simulink model "GPESTN1"  (Simulink 6.1)
settings: Solver=ode45  StartTime=0.0  StopTime=1000.0  MaxStep=0.02  MinStep=0.005  RelTol=1e-3
values from neighbouring files (symbols this model uses):
  A_gpe = 2    [data_GPE.m]    (also in data_GPI.m)
  A_stn = 5    [data_GPI.m]    (also in data_STN.m)
  B_gpe = .08    (= 0.08)    [data_GPE.m]    (also in data_GPI.m)
  B_stn = 1    [data_GPI.m]    (also in data_STN.m)
  c_gpe = 1    [data_GPE.m]
  c_stn = 1    [data_STN.m]
  cag0 = i_v_16(177:192)    [launch_sysGPESTN1.m]    (also in launch_sysGPESTN1_GPEDBS.m)
  cas0 = i_v_16(65:80)    [launch_sysGPESTN1.m]    (also in launch_sysGPESTN1_GPEDBS.m)
  egpegpe = -80    [data_synapses.m]
  egpestn = -100    [data_synapses.m]
  ek_gpe = -80.0    (= -80)    [data_GPE.m]
  ek_stn = -80.0    (= -80)    [data_STN.m]
  el_gpe = -55.0    (= -55)    [data_GPE.m]
  el_stn = -60.0    (= -60)    [data_STN.m]
  epsil_gpe = 1*10^-4    (= 0.0001)    [data_GPE.m]
  epsil_stn = 3.75*10^-5    (= 3.75e-05)    [data_STN.m]
  estngpe = 0    [data_synapses.m]
  gahp_gpe = 30.0    (= 30)    [data_GPE.m]
  gahp_stn = 9.0    (= 9)    [data_STN.m]
  gca_gpe = 0.1    [data_GPE.m]
  gca_stn = 0.5    [data_STN.m]
  ggpegpe = .3    (= 0.3)    [data_synapses.m]    (also in launch_sysGPESTN1.m; launch_sysGPESTN1_GPEDBS.m = 0)
  ggpestn = .90    (= 0.9)    [data_synapses.m]
  gk_gpe = 30.0    (= 30)    [data_GPE.m]
  gk_stn = 45.0    (= 45)    [data_STN.m]
  gl_gpe = .1    (= 0.1)    [data_GPE.m]
  gl_stn = 2.25    [data_STN.m]
  gna_gpe = 120    [data_GPE.m]
  gna_stn = 37.5    [data_STN.m]
  gstngpe = .3    (= 0.3)    [data_synapses.m]
  gt_gpe = .5    (= 0.5)    [data_GPE.m]
  gt_stn = 0.5    [data_STN.m]
  hg0 = i_v_16(129:144)    [launch_sysGPESTN1.m]    (also in launch_sysGPESTN1_GPEDBS.m)
  hs0 = i_v_16(17:32)    [launch_sysGPESTN1.m]    (also in launch_sysGPESTN1_GPEDBS.m)
  k1_gpe = 30.0    (= 30)    [data_GPE.m]
  k1_stn = 15.0    (= 15)    [data_STN.m]
  kca_gpe = 15    [data_GPE.m]
  kca_stn = 22.5    [data_STN.m]
  ng0 = i_v_16(145:160)    [launch_sysGPESTN1.m]    (also in launch_sysGPESTN1_GPEDBS.m)
  ns0 = i_v_16(33:48)    [launch_sysGPESTN1.m]    (also in launch_sysGPESTN1_GPEDBS.m)
  phih_gpe = 0.05    [data_GPE.m]
  phih_stn = 0.75    [data_STN.m]
  phin_gpe = 0.1    [data_GPE.m]
  phin_stn = 0.75    [data_STN.m]
  phir_gpe = 1    [data_GPE.m]
  phir_stn = 0.5    [data_STN.m]
  rg0 = i_v_16(161:176)    [launch_sysGPESTN1.m]    (also in launch_sysGPESTN1_GPEDBS.m)
  rs0 = i_v_16(49:64)    [launch_sysGPESTN1.m]    (also in launch_sysGPESTN1_GPEDBS.m)
  sg0 = i_v_16(193:208)    [launch_sysGPESTN1.m]    (also in launch_sysGPESTN1_GPEDBS.m)
  sigmaa_gpe = 2    [data_GPE.m]
  sigmaa_stn = 7.8    [data_STN.m]
  sigmab_stn = -0.07    [data_STN.m]
  sigmagh_gpe = 2.0    (= 2)    [data_GPE.m]
  sigmagh_stn = 8.0    (= 8)    [data_STN.m]
  sigmah_gpe = -12    [data_GPE.m]
  sigmah_stn = -3.1    [data_STN.m]
  sigmam_gpe = 10.0    (= 10)    [data_GPE.m]
  sigmam_stn = 15.0    (= 15)    [data_STN.m]
  sigman_gpe = 14.0    (= 14)    [data_GPE.m]
  sigman_stn = 8.0    (= 8)    [data_STN.m]
  sigmar_gpe = -2.0    (= -2)    [data_GPE.m]
  sigmar_stn = -2.0    (= -2)    [data_STN.m]
  sigmas_gpe = 2    [data_GPE.m]
  sigmas_stn = 8.0    (= 8)    [data_STN.m]
  sigmatauh_gpe = -12    [data_GPE.m]
  sigmatauh_stn = -3.0    (= -3)    [data_STN.m]
  sigmataun_gpe = -12.0    (= -12)    [data_GPE.m]
  sigmataun_stn = -26.0    (= -26)    [data_STN.m]
  sigmataur_stn = -2.2    [data_STN.m]
  ss0 = i_v_16(81:96)    [launch_sysGPESTN1.m]    (also in launch_sysGPESTN1_GPEDBS.m)
  syn_stngpe_gain = .2    (= 0.2)    [data_STN.m]
  tauh0_gpe = .05    (= 0.05)    [data_GPE.m]
  tauh0_stn = 1.0    (= 1)    [data_STN.m]
  tauh1_gpe = .27    (= 0.27)    [data_GPE.m]
  tauh1_stn = 500.0    (= 500)    [data_STN.m]
  taun0_gpe = .05    (= 0.05)    [data_GPE.m]
  taun0_stn = 1.0    (= 1)    [data_STN.m]
  taun1_gpe = .27    (= 0.27)    [data_GPE.m]
  taun1_stn = 100.0    (= 100)    [data_STN.m]
  taur0_stn = 7.1    [data_STN.m]
  taur1_stn = 17.5    [data_STN.m]
  taur_gpe = 30.0    (= 30)    [data_GPE.m]
  theta_gpe = 20    [data_GPE.m]    (also in data_GPI.m)
  theta_stn = 30    [data_GPI.m]    (also in data_STN.m)
  thetaa_gpe = -57.0    (= -57)    [data_GPE.m]
  thetaa_stn = -63.0    (= -63)    [data_STN.m]
  thetab_stn = 0.25    [data_STN.m]
  thetagh_gpe = -57.0    (= -57)    [data_GPE.m]
  thetagh_stn = -39.0    (= -39)    [data_STN.m]
  thetah_gpe = -58.0    (= -58)    [data_GPE.m]
  thetah_stn = -39.0    (= -39)    [data_STN.m]
  thetam_gpe = -37.0    (= -37)    [data_GPE.m]
  thetam_stn = -30.0    (= -30)    [data_STN.m]
  thetan_gpe = -50.0    (= -50)    [data_GPE.m]
  thetan_stn = -32.0    (= -32)    [data_STN.m]
  thetar_gpe = -70.0    (= -70)    [data_GPE.m]
  thetar_stn = -67.0    (= -67)    [data_STN.m]
  thetas_gpe = -35.0    (= -35)    [data_GPE.m]
  thetas_stn = -39.0    (= -39)    [data_STN.m]
  thetatauh_gpe = -40.0    (= -40)    [data_GPE.m]
  thetatauh_stn = -57.0    (= -57)    [data_STN.m]
  thetataun_gpe = -40.0    (= -40)    [data_GPE.m]
  thetataun_stn = -80.0    (= -80)    [data_STN.m]
  thetataur_stn = 68.0    (= 68)    [data_STN.m]
  vg0 = i_v_16(113:128)    [launch_sysGPESTN1.m]    (also in launch_sysGPESTN1_GPEDBS.m)
  vs0 = i_v_16(1:16)    [launch_sysGPESTN1.m]    (also in launch_sysGPESTN1_GPEDBS.m)
undefined symbols (not defined in the file or in its folder): cag01, cas01, hg01, hs01, ng01, ns01, rg01, rs01, sg01, ss01, vg01, vs01
(part 5 of 9)

== system GPESTN1/STN_cell11/Subsystem/iahp ==
  In1 : Inport  Port=1  LatchInput=off
  In2 : Inport  Port=2  LatchInput=off
  In3 : Inport  Port=3  LatchInput=off
  In4 : Inport  Port=4  LatchInput=off
  Fcn : Fcn  Expr=u/(u+k1_stn)
  Fcn1 : Fcn  Expr=(u-ek_stn)*gahp_stn
  Product : Product  SaturateOnIntegerOverflow=on  InputSameDT=on
  Subsystem : Subsystem
  Out1 : Outport
  wires:
  Subsystem/1(Out1) -> Fcn/1
  Fcn1/1 -> Product/2
  Fcn/1 -> Product/1
  In1/1 -> Subsystem/1(In1)
  In2/1 -> Subsystem/2(In2)
  In3/1 -> Fcn1/1
  Product/1 -> Out1/1
  In4/1 -> Subsystem/3(In3)

== system GPESTN1/STN_cell11/Subsystem/ica ==
  In1 : Inport  Orientation=down  Port=1  LatchInput=off
  ica_stn1 : Subsystem
  sinf : Fcn  Expr=1/(1 + exp(-(u-thetas_stn)/sigmas_stn))
  Out1 : Outport
  wires:
  sinf/1 -> ica_stn1/2(In2)
  In1/1 -> sinf/1, ica_stn1/1(In1)
  ica_stn1/1(Out1) -> Out1/1

== system GPESTN1/STN_cell11/Subsystem/ik ==
  In1 : Inport  Port=1  LatchInput=off
  In2 : Inport  Port=2  LatchInput=off
  ik_stn : Subsystem
  n_stn : Subsystem
  Out1 : Outport
  wires:
  n_stn/1(Out1) -> ik_stn/2(In2)
  In1/1 -> ik_stn/1(In1), n_stn/1(In1)
  ik_stn/1(Out1) -> Out1/1
  In2/1 -> n_stn/2(In2)

== system GPESTN1/STN_cell11/Subsystem/ina ==
  In2 : Inport  Port=1  LatchInput=off
  In1 : Inport  Port=2  LatchInput=off
  h_stn : Subsystem
  ina_stn : Subsystem
  minf : Fcn  Expr=1/(1 + exp(-(u-thetam_stn)/sigmam_stn))
  Out1 : Outport
  wires:
  h_stn/1(Out1) -> ina_stn/3(In3)
  minf/1 -> ina_stn/2(In2)
  In2/1 -> minf/1, h_stn/1(In1), ina_stn/1(In1)
  ina_stn/1(Out1) -> Out1/1
  In1/1 -> h_stn/2(In2)

== system GPESTN1/STN_cell11/Subsystem/it ==
  In2 : Inport  Port=1  LatchInput=off
  In1 : Inport  Port=2  LatchInput=off
  ainf : Fcn  Expr=1/(1 + exp(-(u-thetaa_stn)/sigmaa_stn))
  binf : Fcn  Expr=(1/(1 + exp((u-thetab_stn)/sigmab_stn))) - (1/(1 + exp(-thetab_stn/sigmab_stn)))
  it_stn : Subsystem
  r_stn1 : Subsystem
  Out1 : Outport
  wires:
  ainf/1 -> it_stn/3(In3)
  In2/1 -> r_stn1/1(In1), ainf/1, it_stn/1(In1)
  it_stn/1(Out1) -> Out1/1
  r_stn1/1(Out1) -> binf/1
  binf/1 -> it_stn/2(In2)
  In1/1 -> r_stn1/2(In2)

== system GPESTN1/STN_cell12/Subsystem/iahp ==
  In1 : Inport  Port=1  LatchInput=off
  In2 : Inport  Port=2  LatchInput=off
  In3 : Inport  Port=3  LatchInput=off
  In4 : Inport  Port=4  LatchInput=off
  Fcn : Fcn  Expr=u/(u+k1_stn)
  Fcn1 : Fcn  Expr=(u-ek_stn)*gahp_stn
  Product : Product  SaturateOnIntegerOverflow=on  InputSameDT=on
  Subsystem : Subsystem
  Out1 : Outport
  wires:
  Subsystem/1(Out1) -> Fcn/1
  Fcn1/1 -> Product/2
  Fcn/1 -> Product/1
  In1/1 -> Subsystem/1(In1)
  In2/1 -> Subsystem/2(In2)
  In3/1 -> Fcn1/1
  Product/1 -> Out1/1
  In4/1 -> Subsystem/3(In3)

== system GPESTN1/STN_cell12/Subsystem/ica ==
  In1 : Inport  Orientation=down  Port=1  LatchInput=off
  ica_stn1 : Subsystem
  sinf : Fcn  Expr=1/(1 + exp(-(u-thetas_stn)/sigmas_stn))
  Out1 : Outport
  wires:
  sinf/1 -> ica_stn1/2(In2)
  In1/1 -> sinf/1, ica_stn1/1(In1)
  ica_stn1/1(Out1) -> Out1/1

== system GPESTN1/STN_cell12/Subsystem/ik ==
  In1 : Inport  Port=1  LatchInput=off
  In2 : Inport  Port=2  LatchInput=off
  ik_stn : Subsystem
  n_stn : Subsystem
  Out1 : Outport
  wires:
  n_stn/1(Out1) -> ik_stn/2(In2)
  In1/1 -> ik_stn/1(In1), n_stn/1(In1)
  ik_stn/1(Out1) -> Out1/1
  In2/1 -> n_stn/2(In2)

== system GPESTN1/STN_cell12/Subsystem/ina ==
  In2 : Inport  Port=1  LatchInput=off
  In1 : Inport  Port=2  LatchInput=off
  h_stn : Subsystem
  ina_stn : Subsystem
  minf : Fcn  Expr=1/(1 + exp(-(u-thetam_stn)/sigmam_stn))
  Out1 : Outport
  wires:
  h_stn/1(Out1) -> ina_stn/3(In3)
  minf/1 -> ina_stn/2(In2)
  In2/1 -> minf/1, h_stn/1(In1), ina_stn/1(In1)
  ina_stn/1(Out1) -> Out1/1
  In1/1 -> h_stn/2(In2)

== system GPESTN1/STN_cell12/Subsystem/it ==
  In2 : Inport  Port=1  LatchInput=off
  In1 : Inport  Port=2  LatchInput=off
  ainf : Fcn  Expr=1/(1 + exp(-(u-thetaa_stn)/sigmaa_stn))
  binf : Fcn  Expr=(1/(1 + exp((u-thetab_stn)/sigmab_stn))) - (1/(1 + exp(-thetab_stn/sigmab_stn)))
  it_stn : Subsystem
  r_stn1 : Subsystem
  Out1 : Outport
  wires:
  ainf/1 -> it_stn/3(In3)
  In2/1 -> r_stn1/1(In1), ainf/1, it_stn/1(In1)
  it_stn/1(Out1) -> Out1/1
  r_stn1/1(Out1) -> binf/1
  binf/1 -> it_stn/2(In2)
  In1/1 -> r_stn1/2(In2)

== system GPESTN1/STN_cell13/Subsystem/iahp ==
  In1 : Inport  Port=1  LatchInput=off
  In2 : Inport  Port=2  LatchInput=off
  In3 : Inport  Port=3  LatchInput=off
  In4 : Inport  Port=4  LatchInput=off
  Fcn : Fcn  Expr=u/(u+k1_stn)
  Fcn1 : Fcn  Expr=(u-ek_stn)*gahp_stn
  Product : Product  SaturateOnIntegerOverflow=on  InputSameDT=on
  Subsystem : Subsystem
  Out1 : Outport
  wires:
  Subsystem/1(Out1) -> Fcn/1
  Fcn1/1 -> Product/2
  Fcn/1 -> Product/1
  In1/1 -> Subsystem/1(In1)
  In2/1 -> Subsystem/2(In2)
  In3/1 -> Fcn1/1
  Product/1 -> Out1/1
  In4/1 -> Subsystem/3(In3)

== system GPESTN1/STN_cell13/Subsystem/ica ==
  In1 : Inport  Orientation=down  Port=1  LatchInput=off
  ica_stn1 : Subsystem
  sinf : Fcn  Expr=1/(1 + exp(-(u-thetas_stn)/sigmas_stn))
  Out1 : Outport
  wires:
  sinf/1 -> ica_stn1/2(In2)
  In1/1 -> sinf/1, ica_stn1/1(In1)
  ica_stn1/1(Out1) -> Out1/1

== system GPESTN1/STN_cell13/Subsystem/ik ==
  In1 : Inport  Port=1  LatchInput=off
  In2 : Inport  Port=2  LatchInput=off
  ik_stn : Subsystem
  n_stn : Subsystem
  Out1 : Outport
  wires:
  n_stn/1(Out1) -> ik_stn/2(In2)
  In1/1 -> ik_stn/1(In1), n_stn/1(In1)
  ik_stn/1(Out1) -> Out1/1
  In2/1 -> n_stn/2(In2)

== system GPESTN1/STN_cell13/Subsystem/ina ==
  In2 : Inport  Port=1  LatchInput=off
  In1 : Inport  Port=2  LatchInput=off
  h_stn : Subsystem
  ina_stn : Subsystem
  minf : Fcn  Expr=1/(1 + exp(-(u-thetam_stn)/sigmam_stn))
  Out1 : Outport
  wires:
  h_stn/1(Out1) -> ina_stn/3(In3)
  minf/1 -> ina_stn/2(In2)
  In2/1 -> minf/1, h_stn/1(In1), ina_stn/1(In1)
  ina_stn/1(Out1) -> Out1/1
  In1/1 -> h_stn/2(In2)

== system GPESTN1/STN_cell13/Subsystem/it ==
  In2 : Inport  Port=1  LatchInput=off
  In1 : Inport  Port=2  LatchInput=off
  ainf : Fcn  Expr=1/(1 + exp(-(u-thetaa_stn)/sigmaa_stn))
  binf : Fcn  Expr=(1/(1 + exp((u-thetab_stn)/sigmab_stn))) - (1/(1 + exp(-thetab_stn/sigmab_stn)))
  it_stn : Subsystem
  r_stn1 : Subsystem
  Out1 : Outport
  wires:
  ainf/1 -> it_stn/3(In3)
  In2/1 -> r_stn1/1(In1), ainf/1, it_stn/1(In1)
  it_stn/1(Out1) -> Out1/1
  r_stn1/1(Out1) -> binf/1
  binf/1 -> it_stn/2(In2)
  In1/1 -> r_stn1/2(In2)

== system GPESTN1/STN_cell14/Subsystem/iahp ==
  In1 : Inport  Port=1  LatchInput=off
  In2 : Inport  Port=2  LatchInput=off
  In3 : Inport  Port=3  LatchInput=off
  In4 : Inport  Port=4  LatchInput=off
  Fcn : Fcn  Expr=u/(u+k1_stn)
  Fcn1 : Fcn  Expr=(u-ek_stn)*gahp_stn
  Product : Product  SaturateOnIntegerOverflow=on  InputSameDT=on
  Subsystem : Subsystem
  Out1 : Outport
  wires:
  Subsystem/1(Out1) -> Fcn/1
  Fcn1/1 -> Product/2
  Fcn/1 -> Product/1
  In1/1 -> Subsystem/1(In1)
  In2/1 -> Subsystem/2(In2)
  In3/1 -> Fcn1/1
  Product/1 -> Out1/1
  In4/1 -> Subsystem/3(In3)

== system GPESTN1/STN_cell14/Subsystem/ica ==
  In1 : Inport  Orientation=down  Port=1  LatchInput=off
  ica_stn1 : Subsystem
  sinf : Fcn  Expr=1/(1 + exp(-(u-thetas_stn)/sigmas_stn))
  Out1 : Outport
  wires:
  sinf/1 -> ica_stn1/2(In2)
  In1/1 -> sinf/1, ica_stn1/1(In1)
  ica_stn1/1(Out1) -> Out1/1

== system GPESTN1/STN_cell14/Subsystem/ik ==
  In1 : Inport  Port=1  LatchInput=off
  In2 : Inport  Port=2  LatchInput=off
  ik_stn : Subsystem
  n_stn : Subsystem
  Out1 : Outport
  wires:
  n_stn/1(Out1) -> ik_stn/2(In2)
  In1/1 -> ik_stn/1(In1), n_stn/1(In1)
  ik_stn/1(Out1) -> Out1/1
  In2/1 -> n_stn/2(In2)

== system GPESTN1/STN_cell14/Subsystem/ina ==
  In2 : Inport  Port=1  LatchInput=off
  In1 : Inport  Port=2  LatchInput=off
  h_stn : Subsystem
  ina_stn : Subsystem
  minf : Fcn  Expr=1/(1 + exp(-(u-thetam_stn)/sigmam_stn))
  Out1 : Outport
  wires:
  h_stn/1(Out1) -> ina_stn/3(In3)
  minf/1 -> ina_stn/2(In2)
  In2/1 -> minf/1, h_stn/1(In1), ina_stn/1(In1)
  ina_stn/1(Out1) -> Out1/1
  In1/1 -> h_stn/2(In2)

== system GPESTN1/STN_cell14/Subsystem/it ==
  In2 : Inport  Port=1  LatchInput=off
  In1 : Inport  Port=2  LatchInput=off
  ainf : Fcn  Expr=1/(1 + exp(-(u-thetaa_stn)/sigmaa_stn))
  binf : Fcn  Expr=(1/(1 + exp((u-thetab_stn)/sigmab_stn))) - (1/(1 + exp(-thetab_stn/sigmab_stn)))
  it_stn : Subsystem
  r_stn1 : Subsystem
  Out1 : Outport
  wires:
  ainf/1 -> it_stn/3(In3)
  In2/1 -> r_stn1/1(In1), ainf/1, it_stn/1(In1)
  it_stn/1(Out1) -> Out1/1
  r_stn1/1(Out1) -> binf/1
  binf/1 -> it_stn/2(In2)
  In1/1 -> r_stn1/2(In2)

== system GPESTN1/STN_cell15/Subsystem/iahp ==
  In1 : Inport  Port=1  LatchInput=off
  In2 : Inport  Port=2  LatchInput=off
  In3 : Inport  Port=3  LatchInput=off
  In4 : Inport  Port=4  LatchInput=off
  Fcn : Fcn  Expr=u/(u+k1_stn)
  Fcn1 : Fcn  Expr=(u-ek_stn)*gahp_stn
  Product : Product  SaturateOnIntegerOverflow=on  InputSameDT=on
  Subsystem : Subsystem
  Out1 : Outport
  wires:
  Subsystem/1(Out1) -> Fcn/1
  Fcn1/1 -> Product/2
  Fcn/1 -> Product/1
  In1/1 -> Subsystem/1(In1)
  In2/1 -> Subsystem/2(In2)
  In3/1 -> Fcn1/1
  Product/1 -> Out1/1
  In4/1 -> Subsystem/3(In3)

== system GPESTN1/STN_cell15/Subsystem/ica ==
  In1 : Inport  Orientation=down  Port=1  LatchInput=off
  ica_stn1 : Subsystem
  sinf : Fcn  Expr=1/(1 + exp(-(u-thetas_stn)/sigmas_stn))
  Out1 : Outport
  wires:
  sinf/1 -> ica_stn1/2(In2)
  In1/1 -> sinf/1, ica_stn1/1(In1)
  ica_stn1/1(Out1) -> Out1/1

== system GPESTN1/STN_cell15/Subsystem/ik ==
  In1 : Inport  Port=1  LatchInput=off
  In2 : Inport  Port=2  LatchInput=off
  ik_stn : Subsystem
  n_stn : Subsystem
  Out1 : Outport
  wires:
  n_stn/1(Out1) -> ik_stn/2(In2)
  In1/1 -> ik_stn/1(In1), n_stn/1(In1)
  ik_stn/1(Out1) -> Out1/1
  In2/1 -> n_stn/2(In2)

== system GPESTN1/STN_cell15/Subsystem/ina ==
  In2 : Inport  Port=1  LatchInput=off
  In1 : Inport  Port=2  LatchInput=off
  h_stn : Subsystem
  ina_stn : Subsystem
  minf : Fcn  Expr=1/(1 + exp(-(u-thetam_stn)/sigmam_stn))
  Out1 : Outport
  wires:
  h_stn/1(Out1) -> ina_stn/3(In3)
  minf/1 -> ina_stn/2(In2)
  In2/1 -> minf/1, h_stn/1(In1), ina_stn/1(In1)
  ina_stn/1(Out1) -> Out1/1
  In1/1 -> h_stn/2(In2)

== system GPESTN1/STN_cell15/Subsystem/it ==
  In2 : Inport  Port=1  LatchInput=off
  In1 : Inport  Port=2  LatchInput=off
  ainf : Fcn  Expr=1/(1 + exp(-(u-thetaa_stn)/sigmaa_stn))
  binf : Fcn  Expr=(1/(1 + exp((u-thetab_stn)/sigmab_stn))) - (1/(1 + exp(-thetab_stn/sigmab_stn)))
  it_stn : Subsystem
  r_stn1 : Subsystem
  Out1 : Outport
  wires:
  ainf/1 -> it_stn/3(In3)
  In2/1 -> r_stn1/1(In1), ainf/1, it_stn/1(In1)
  it_stn/1(Out1) -> Out1/1
  r_stn1/1(Out1) -> binf/1
  binf/1 -> it_stn/2(In2)
  In1/1 -> r_stn1/2(In2)

== system GPESTN1/STN_cell16/Subsystem/iahp ==
  In1 : Inport  Port=1  LatchInput=off
  In2 : Inport  Port=2  LatchInput=off
  In3 : Inport  Port=3  LatchInput=off
  In4 : Inport  Port=4  LatchInput=off
  Fcn : Fcn  Expr=u/(u+k1_stn)
  Fcn1 : Fcn  Expr=(u-ek_stn)*gahp_stn
  Product : Product  SaturateOnIntegerOverflow=on  InputSameDT=on
  Subsystem : Subsystem
  Out1 : Outport
  wires:
  Subsystem/1(Out1) -> Fcn/1
  Fcn1/1 -> Product/2
  Fcn/1 -> Product/1
  In1/1 -> Subsystem/1(In1)
  In2/1 -> Subsystem/2(In2)
  In3/1 -> Fcn1/1
  Product/1 -> Out1/1
  In4/1 -> Subsystem/3(In3)

== system GPESTN1/STN_cell16/Subsystem/ica ==
  In1 : Inport  Orientation=down  Port=1  LatchInput=off
  ica_stn1 : Subsystem
  sinf : Fcn  Expr=1/(1 + exp(-(u-thetas_stn)/sigmas_stn))
  Out1 : Outport
  wires:
  sinf/1 -> ica_stn1/2(In2)
  In1/1 -> sinf/1, ica_stn1/1(In1)
  ica_stn1/1(Out1) -> Out1/1

== system GPESTN1/STN_cell16/Subsystem/ik ==
  In1 : Inport  Port=1  LatchInput=off
  In2 : Inport  Port=2  LatchInput=off
  ik_stn : Subsystem
  n_stn : Subsystem
  Out1 : Outport
  wires:
  n_stn/1(Out1) -> ik_stn/2(In2)
  In1/1 -> ik_stn/1(In1), n_stn/1(In1)
  ik_stn/1(Out1) -> Out1/1
  In2/1 -> n_stn/2(In2)

== system GPESTN1/STN_cell16/Subsystem/ina ==
  In2 : Inport  Port=1  LatchInput=off
  In1 : Inport  Port=2  LatchInput=off
  h_stn : Subsystem
  ina_stn : Subsystem
  minf : Fcn  Expr=1/(1 + exp(-(u-thetam_stn)/sigmam_stn))
  Out1 : Outport
  wires:
  h_stn/1(Out1) -> ina_stn/3(In3)
  minf/1 -> ina_stn/2(In2)
  In2/1 -> minf/1, h_stn/1(In1), ina_stn/1(In1)
  ina_stn/1(Out1) -> Out1/1
  In1/1 -> h_stn/2(In2)

== system GPESTN1/STN_cell16/Subsystem/it ==
  In2 : Inport  Port=1  LatchInput=off
  In1 : Inport  Port=2  LatchInput=off
  ainf : Fcn  Expr=1/(1 + exp(-(u-thetaa_stn)/sigmaa_stn))
  binf : Fcn  Expr=(1/(1 + exp((u-thetab_stn)/sigmab_stn))) - (1/(1 + exp(-thetab_stn/sigmab_stn)))
  it_stn : Subsystem
  r_stn1 : Subsystem
  Out1 : Outport
  wires:
  ainf/1 -> it_stn/3(In3)
  In2/1 -> r_stn1/1(In1), ainf/1, it_stn/1(In1)
  it_stn/1(Out1) -> Out1/1
  r_stn1/1(Out1) -> binf/1
  binf/1 -> it_stn/2(In2)
  In1/1 -> r_stn1/2(In2)

== system GPESTN1/STN_cell17/Subsystem/iahp ==
  In1 : Inport  Port=1  LatchInput=off
  In2 : Inport  Port=2  LatchInput=off
  In3 : Inport  Port=3  LatchInput=off
  In4 : Inport  Port=4  LatchInput=off
  Fcn : Fcn  Expr=u/(u+k1_stn)
  Fcn1 : Fcn  Expr=(u-ek_stn)*gahp_stn
  Product : Product  SaturateOnIntegerOverflow=on  InputSameDT=on
  Subsystem : Subsystem
  Out1 : Outport
  wires:
  Subsystem/1(Out1) -> Fcn/1
  Fcn1/1 -> Product/2
  Fcn/1 -> Product/1
  In1/1 -> Subsystem/1(In1)
  In2/1 -> Subsystem/2(In2)
  In3/1 -> Fcn1/1
  Product/1 -> Out1/1
  In4/1 -> Subsystem/3(In3)

== system GPESTN1/STN_cell17/Subsystem/ica ==
  In1 : Inport  Orientation=down  Port=1  LatchInput=off
  ica_stn1 : Subsystem
  sinf : Fcn  Expr=1/(1 + exp(-(u-thetas_stn)/sigmas_stn))
  Out1 : Outport
  wires:
  sinf/1 -> ica_stn1/2(In2)
  In1/1 -> sinf/1, ica_stn1/1(In1)
  ica_stn1/1(Out1) -> Out1/1

== system GPESTN1/STN_cell17/Subsystem/ik ==
  In1 : Inport  Port=1  LatchInput=off
  In2 : Inport  Port=2  LatchInput=off
  ik_stn : Subsystem
  n_stn : Subsystem
  Out1 : Outport
  wires:
  n_stn/1(Out1) -> ik_stn/2(In2)
  In1/1 -> ik_stn/1(In1), n_stn/1(In1)
  ik_stn/1(Out1) -> Out1/1
  In2/1 -> n_stn/2(In2)

== system GPESTN1/STN_cell17/Subsystem/ina ==
  In2 : Inport  Port=1  LatchInput=off
  In1 : Inport  Port=2  LatchInput=off
  h_stn : Subsystem
  ina_stn : Subsystem
  minf : Fcn  Expr=1/(1 + exp(-(u-thetam_stn)/sigmam_stn))
  Out1 : Outport
  wires:
  h_stn/1(Out1) -> ina_stn/3(In3)
  minf/1 -> ina_stn/2(In2)
  In2/1 -> minf/1, h_stn/1(In1), ina_stn/1(In1)
  ina_stn/1(Out1) -> Out1/1
  In1/1 -> h_stn/2(In2)

== system GPESTN1/STN_cell17/Subsystem/it ==
  In2 : Inport  Port=1  LatchInput=off
  In1 : Inport  Port=2  LatchInput=off
  ainf : Fcn  Expr=1/(1 + exp(-(u-thetaa_stn)/sigmaa_stn))
  binf : Fcn  Expr=(1/(1 + exp((u-thetab_stn)/sigmab_stn))) - (1/(1 + exp(-thetab_stn/sigmab_stn)))
  it_stn : Subsystem
  r_stn1 : Subsystem
  Out1 : Outport
  wires:
  ainf/1 -> it_stn/3(In3)
  In2/1 -> r_stn1/1(In1), ainf/1, it_stn/1(In1)
  it_stn/1(Out1) -> Out1/1
  r_stn1/1(Out1) -> binf/1
  binf/1 -> it_stn/2(In2)
  In1/1 -> r_stn1/2(In2)

== system GPESTN1/STN_cell2/Subsystem/iahp ==
  In1 : Inport  Port=1  LatchInput=off
  In2 : Inport  Port=2  LatchInput=off
  In3 : Inport  Port=3  LatchInput=off
  In4 : Inport  Port=4  LatchInput=off
  Fcn : Fcn  Expr=u/(u+k1_stn)
  Fcn1 : Fcn  Expr=(u-ek_stn)*gahp_stn
  Product : Product  SaturateOnIntegerOverflow=on  InputSameDT=on
  Subsystem : Subsystem
  Out1 : Outport
  wires:
  Subsystem/1(Out1) -> Fcn/1
  Fcn1/1 -> Product/2
  Fcn/1 -> Product/1
  In1/1 -> Subsystem/1(In1)
  In2/1 -> Subsystem/2(In2)
  In3/1 -> Fcn1/1
  Product/1 -> Out1/1
  In4/1 -> Subsystem/3(In3)

== system GPESTN1/STN_cell2/Subsystem/ica ==
  In1 : Inport  Orientation=down  Port=1  LatchInput=off
  ica_stn1 : Subsystem
  sinf : Fcn  Expr=1/(1 + exp(-(u-thetas_stn)/sigmas_stn))
  Out1 : Outport
  wires:
  sinf/1 -> ica_stn1/2(In2)
  In1/1 -> sinf/1, ica_stn1/1(In1)
  ica_stn1/1(Out1) -> Out1/1

== system GPESTN1/STN_cell2/Subsystem/ik ==
  In1 : Inport  Port=1  LatchInput=off
  In2 : Inport  Port=2  LatchInput=off
  ik_stn : Subsystem
  n_stn : Subsystem
  Out1 : Outport
  wires:
  n_stn/1(Out1) -> ik_stn/2(In2)
  In1/1 -> ik_stn/1(In1), n_stn/1(In1)
  ik_stn/1(Out1) -> Out1/1
  In2/1 -> n_stn/2(In2)

== system GPESTN1/STN_cell2/Subsystem/ina ==
  In2 : Inport  Port=1  LatchInput=off
  In1 : Inport  Port=2  LatchInput=off
  h_stn : Subsystem
  ina_stn : Subsystem
  minf : Fcn  Expr=1/(1 + exp(-(u-thetam_stn)/sigmam_stn))
  Out1 : Outport
  wires:
  h_stn/1(Out1) -> ina_stn/3(In3)
  minf/1 -> ina_stn/2(In2)
  In2/1 -> minf/1, h_stn/1(In1), ina_stn/1(In1)
  ina_stn/1(Out1) -> Out1/1
  In1/1 -> h_stn/2(In2)

== system GPESTN1/STN_cell2/Subsystem/it ==
  In2 : Inport  Port=1  LatchInput=off
  In1 : Inport  Port=2  LatchInput=off
  ainf : Fcn  Expr=1/(1 + exp(-(u-thetaa_stn)/sigmaa_stn))
  binf : Fcn  Expr=(1/(1 + exp((u-thetab_stn)/sigmab_stn))) - (1/(1 + exp(-thetab_stn/sigmab_stn)))
  it_stn : Subsystem
  r_stn1 : Subsystem
  Out1 : Outport
  wires:
  ainf/1 -> it_stn/3(In3)
  In2/1 -> r_stn1/1(In1), ainf/1, it_stn/1(In1)
  it_stn/1(Out1) -> Out1/1
  r_stn1/1(Out1) -> binf/1
  binf/1 -> it_stn/2(In2)
  In1/1 -> r_stn1/2(In2)

== system GPESTN1/STN_cell3/Subsystem/iahp ==
  In1 : Inport  Port=1  LatchInput=off
  In2 : Inport  Port=2  LatchInput=off
  In3 : Inport  Port=3  LatchInput=off
  In4 : Inport  Port=4  LatchInput=off
  Fcn : Fcn  Expr=u/(u+k1_stn)
  Fcn1 : Fcn  Expr=(u-ek_stn)*gahp_stn
  Product : Product  SaturateOnIntegerOverflow=on  InputSameDT=on
  Subsystem : Subsystem
  Out1 : Outport
  wires:
  Subsystem/1(Out1) -> Fcn/1
  Fcn1/1 -> Product/2
  Fcn/1 -> Product/1
  In1/1 -> Subsystem/1(In1)
  In2/1 -> Subsystem/2(In2)
  In3/1 -> Fcn1/1
  Product/1 -> Out1/1
  In4/1 -> Subsystem/3(In3)

== system GPESTN1/STN_cell3/Subsystem/ica ==
  In1 : Inport  Orientation=down  Port=1  LatchInput=off
  ica_stn1 : Subsystem
  sinf : Fcn  Expr=1/(1 + exp(-(u-thetas_stn)/sigmas_stn))
  Out1 : Outport
  wires:
  sinf/1 -> ica_stn1/2(In2)
  In1/1 -> sinf/1, ica_stn1/1(In1)
  ica_stn1/1(Out1) -> Out1/1

== system GPESTN1/STN_cell3/Subsystem/ik ==
  In1 : Inport  Port=1  LatchInput=off
  In2 : Inport  Port=2  LatchInput=off
  ik_stn : Subsystem
  n_stn : Subsystem
  Out1 : Outport
  wires:
  n_stn/1(Out1) -> ik_stn/2(In2)
  In1/1 -> ik_stn/1(In1), n_stn/1(In1)
  ik_stn/1(Out1) -> Out1/1
  In2/1 -> n_stn/2(In2)

== system GPESTN1/STN_cell3/Subsystem/ina ==
  In2 : Inport  Port=1  LatchInput=off
  In1 : Inport  Port=2  LatchInput=off
  h_stn : Subsystem
  ina_stn : Subsystem
  minf : Fcn  Expr=1/(1 + exp(-(u-thetam_stn)/sigmam_stn))
  Out1 : Outport
  wires:
  h_stn/1(Out1) -> ina_stn/3(In3)
  minf/1 -> ina_stn/2(In2)
  In2/1 -> minf/1, h_stn/1(In1), ina_stn/1(In1)
  ina_stn/1(Out1) -> Out1/1
  In1/1 -> h_stn/2(In2)

== system GPESTN1/STN_cell3/Subsystem/it ==
  In2 : Inport  Port=1  LatchInput=off
  In1 : Inport  Port=2  LatchInput=off
  ainf : Fcn  Expr=1/(1 + exp(-(u-thetaa_stn)/sigmaa_stn))
  binf : Fcn  Expr=(1/(1 + exp((u-thetab_stn)/sigmab_stn))) - (1/(1 + exp(-thetab_stn/sigmab_stn)))
  it_stn : Subsystem
  r_stn1 : Subsystem
  Out1 : Outport
  wires:
  ainf/1 -> it_stn/3(In3)
  In2/1 -> r_stn1/1(In1), ainf/1, it_stn/1(In1)
  it_stn/1(Out1) -> Out1/1
  r_stn1/1(Out1) -> binf/1
  binf/1 -> it_stn/2(In2)
  In1/1 -> r_stn1/2(In2)

== system GPESTN1/STN_cell5/Subsystem/iahp ==
  In1 : Inport  Port=1  LatchInput=off
  In2 : Inport  Port=2  LatchInput=off
  In3 : Inport  Port=3  LatchInput=off
  In4 : Inport  Port=4  LatchInput=off
  Fcn : Fcn  Expr=u/(u+k1_stn)
  Fcn1 : Fcn  Expr=(u-ek_stn)*gahp_stn
  Product : Product  SaturateOnIntegerOverflow=on  InputSameDT=on
  Subsystem : Subsystem
  Out1 : Outport
  wires:
  Subsystem/1(Out1) -> Fcn/1
  Fcn1/1 -> Product/2
  Fcn/1 -> Product/1
  In1/1 -> Subsystem/1(In1)
  In2/1 -> Subsystem/2(In2)
  In3/1 -> Fcn1/1
  Product/1 -> Out1/1
  In4/1 -> Subsystem/3(In3)

== system GPESTN1/STN_cell5/Subsystem/ica ==
  In1 : Inport  Orientation=down  Port=1  LatchInput=off
  ica_stn1 : Subsystem
  sinf : Fcn  Expr=1/(1 + exp(-(u-thetas_stn)/sigmas_stn))
  Out1 : Outport
  wires:
  sinf/1 -> ica_stn1/2(In2)
  In1/1 -> sinf/1, ica_stn1/1(In1)
  ica_stn1/1(Out1) -> Out1/1

== system GPESTN1/STN_cell5/Subsystem/ik ==
  In1 : Inport  Port=1  LatchInput=off
  In2 : Inport  Port=2  LatchInput=off
  ik_stn : Subsystem
  n_stn : Subsystem
  Out1 : Outport
  wires:
  n_stn/1(Out1) -> ik_stn/2(In2)
  In1/1 -> ik_stn/1(In1), n_stn/1(In1)
  ik_stn/1(Out1) -> Out1/1
  In2/1 -> n_stn/2(In2)

== system GPESTN1/STN_cell5/Subsystem/ina ==
  In2 : Inport  Port=1  LatchInput=off
  In1 : Inport  Port=2  LatchInput=off
  h_stn : Subsystem
  ina_stn : Subsystem
  minf : Fcn  Expr=1/(1 + exp(-(u-thetam_stn)/sigmam_stn))
  Out1 : Outport
  wires:
  h_stn/1(Out1) -> ina_stn/3(In3)
  minf/1 -> ina_stn/2(In2)
  In2/1 -> minf/1, h_stn/1(In1), ina_stn/1(In1)
  ina_stn/1(Out1) -> Out1/1
  In1/1 -> h_stn/2(In2)

== system GPESTN1/STN_cell5/Subsystem/it ==
  In2 : Inport  Port=1  LatchInput=off
  In1 : Inport  Port=2  LatchInput=off
  ainf : Fcn  Expr=1/(1 + exp(-(u-thetaa_stn)/sigmaa_stn))
  binf : Fcn  Expr=(1/(1 + exp((u-thetab_stn)/sigmab_stn))) - (1/(1 + exp(-thetab_stn/sigmab_stn)))
  it_stn : Subsystem
  r_stn1 : Subsystem
  Out1 : Outport
  wires:
  ainf/1 -> it_stn/3(In3)
  In2/1 -> r_stn1/1(In1), ainf/1, it_stn/1(In1)
  it_stn/1(Out1) -> Out1/1
  r_stn1/1(Out1) -> binf/1
  binf/1 -> it_stn/2(In2)
  In1/1 -> r_stn1/2(In2)

== system GPESTN1/STN_cell6/Subsystem/iahp ==
  In1 : Inport  Port=1  LatchInput=off
  In2 : Inport  Port=2  LatchInput=off
  In3 : Inport  Port=3  LatchInput=off
  In4 : Inport  Port=4  LatchInput=off
  Fcn : Fcn  Expr=u/(u+k1_stn)
  Fcn1 : Fcn  Expr=(u-ek_stn)*gahp_stn
  Product : Product  SaturateOnIntegerOverflow=on  InputSameDT=on
  Subsystem : Subsystem
  Out1 : Outport
  wires:
  Subsystem/1(Out1) -> Fcn/1
  Fcn1/1 -> Product/2
  Fcn/1 -> Product/1
  In1/1 -> Subsystem/1(In1)
  In2/1 -> Subsystem/2(In2)
  In3/1 -> Fcn1/1
  Product/1 -> Out1/1
  In4/1 -> Subsystem/3(In3)

== system GPESTN1/STN_cell6/Subsystem/ica ==
  In1 : Inport  Orientation=down  Port=1  LatchInput=off
  ica_stn1 : Subsystem
  sinf : Fcn  Expr=1/(1 + exp(-(u-thetas_stn)/sigmas_stn))
  Out1 : Outport
  wires:
  sinf/1 -> ica_stn1/2(In2)
  In1/1 -> sinf/1, ica_stn1/1(In1)
  ica_stn1/1(Out1) -> Out1/1

== system GPESTN1/STN_cell6/Subsystem/ik ==
  In1 : Inport  Port=1  LatchInput=off
  In2 : Inport  Port=2  LatchInput=off
  ik_stn : Subsystem
  n_stn : Subsystem
  Out1 : Outport
  wires:
  n_stn/1(Out1) -> ik_stn/2(In2)
  In1/1 -> ik_stn/1(In1), n_stn/1(In1)
  ik_stn/1(Out1) -> Out1/1
  In2/1 -> n_stn/2(In2)

== system GPESTN1/STN_cell6/Subsystem/ina ==
  In2 : Inport  Port=1  LatchInput=off
  In1 : Inport  Port=2  LatchInput=off
  h_stn : Subsystem
  ina_stn : Subsystem
  minf : Fcn  Expr=1/(1 + exp(-(u-thetam_stn)/sigmam_stn))
  Out1 : Outport
  wires:
  h_stn/1(Out1) -> ina_stn/3(In3)
  minf/1 -> ina_stn/2(In2)
  In2/1 -> minf/1, h_stn/1(In1), ina_stn/1(In1)
  ina_stn/1(Out1) -> Out1/1
  In1/1 -> h_stn/2(In2)

== system GPESTN1/STN_cell6/Subsystem/it ==
  In2 : Inport  Port=1  LatchInput=off
  In1 : Inport  Port=2  LatchInput=off
  ainf : Fcn  Expr=1/(1 + exp(-(u-thetaa_stn)/sigmaa_stn))
  binf : Fcn  Expr=(1/(1 + exp((u-thetab_stn)/sigmab_stn))) - (1/(1 + exp(-thetab_stn/sigmab_stn)))
  it_stn : Subsystem
  r_stn1 : Subsystem
  Out1 : Outport
  wires:
  ainf/1 -> it_stn/3(In3)
  In2/1 -> r_stn1/1(In1), ainf/1, it_stn/1(In1)
  it_stn/1(Out1) -> Out1/1
  r_stn1/1(Out1) -> binf/1
  binf/1 -> it_stn/2(In2)
  In1/1 -> r_stn1/2(In2)

== system GPESTN1/STN_cell7/Subsystem/iahp ==
  In1 : Inport  Port=1  LatchInput=off
  In2 : Inport  Port=2  LatchInput=off
  In3 : Inport  Port=3  LatchInput=off
  In4 : Inport  Port=4  LatchInput=off
  Fcn : Fcn  Expr=u/(u+k1_stn)
  Fcn1 : Fcn  Expr=(u-ek_stn)*gahp_stn
  Product : Product  SaturateOnIntegerOverflow=on  InputSameDT=on
  Subsystem : Subsystem
  Out1 : Outport
  wires:
  Subsystem/1(Out1) -> Fcn/1
  Fcn1/1 -> Product/2
  Fcn/1 -> Product/1
  In1/1 -> Subsystem/1(In1)
  In2/1 -> Subsystem/2(In2)
  In3/1 -> Fcn1/1
  Product/1 -> Out1/1
  In4/1 -> Subsystem/3(In3)

== system GPESTN1/STN_cell7/Subsystem/ica ==
  In1 : Inport  Orientation=down  Port=1  LatchInput=off
  ica_stn1 : Subsystem
  sinf : Fcn  Expr=1/(1 + exp(-(u-thetas_stn)/sigmas_stn))
  Out1 : Outport
  wires:
  sinf/1 -> ica_stn1/2(In2)
  In1/1 -> sinf/1, ica_stn1/1(In1)
  ica_stn1/1(Out1) -> Out1/1

== system GPESTN1/STN_cell7/Subsystem/ik ==
  In1 : Inport  Port=1  LatchInput=off
  In2 : Inport  Port=2  LatchInput=off
  ik_stn : Subsystem
  n_stn : Subsystem
  Out1 : Outport
  wires:
  n_stn/1(Out1) -> ik_stn/2(In2)
  In1/1 -> ik_stn/1(In1), n_stn/1(In1)
  ik_stn/1(Out1) -> Out1/1
  In2/1 -> n_stn/2(In2)

== system GPESTN1/STN_cell7/Subsystem/ina ==
  In2 : Inport  Port=1  LatchInput=off
  In1 : Inport  Port=2  LatchInput=off
  h_stn : Subsystem
  ina_stn : Subsystem
  minf : Fcn  Expr=1/(1 + exp(-(u-thetam_stn)/sigmam_stn))
  Out1 : Outport
  wires:
  h_stn/1(Out1) -> ina_stn/3(In3)
  minf/1 -> ina_stn/2(In2)
  In2/1 -> minf/1, h_stn/1(In1), ina_stn/1(In1)
  ina_stn/1(Out1) -> Out1/1
  In1/1 -> h_stn/2(In2)

== system GPESTN1/STN_cell7/Subsystem/it ==
  In2 : Inport  Port=1  LatchInput=off
  In1 : Inport  Port=2  LatchInput=off
  ainf : Fcn  Expr=1/(1 + exp(-(u-thetaa_stn)/sigmaa_stn))
  binf : Fcn  Expr=(1/(1 + exp((u-thetab_stn)/sigmab_stn))) - (1/(1 + exp(-thetab_stn/sigmab_stn)))
  it_stn : Subsystem
  r_stn1 : Subsystem
  Out1 : Outport
  wires:
  ainf/1 -> it_stn/3(In3)
  In2/1 -> r_stn1/1(In1), ainf/1, it_stn/1(In1)
  it_stn/1(Out1) -> Out1/1
  r_stn1/1(Out1) -> binf/1
  binf/1 -> it_stn/2(In2)
  In1/1 -> r_stn1/2(In2)

== system GPESTN1/STN_cell8/Subsystem/iahp ==
  In1 : Inport  Port=1  LatchInput=off
  In2 : Inport  Port=2  LatchInput=off
  In3 : Inport  Port=3  LatchInput=off
  In4 : Inport  Port=4  LatchInput=off
  Fcn : Fcn  Expr=u/(u+k1_stn)
  Fcn1 : Fcn  Expr=(u-ek_stn)*gahp_stn
  Product : Product  SaturateOnIntegerOverflow=on  InputSameDT=on
  Subsystem : Subsystem
  Out1 : Outport
  wires:
  Subsystem/1(Out1) -> Fcn/1
  Fcn1/1 -> Product/2
  Fcn/1 -> Product/1
  In1/1 -> Subsystem/1(In1)
  In2/1 -> Subsystem/2(In2)
  In3/1 -> Fcn1/1
  Product/1 -> Out1/1
  In4/1 -> Subsystem/3(In3)

== system GPESTN1/STN_cell8/Subsystem/ica ==
  In1 : Inport  Orientation=down  Port=1  LatchInput=off
  ica_stn1 : Subsystem
  sinf : Fcn  Expr=1/(1 + exp(-(u-thetas_stn)/sigmas_stn))
  Out1 : Outport
  wires:
  sinf/1 -> ica_stn1/2(In2)
  In1/1 -> sinf/1, ica_stn1/1(In1)
  ica_stn1/1(Out1) -> Out1/1

== system GPESTN1/STN_cell8/Subsystem/ik ==
  In1 : Inport  Port=1  LatchInput=off
  In2 : Inport  Port=2  LatchInput=off
  ik_stn : Subsystem
  n_stn : Subsystem
  Out1 : Outport
  wires:
  n_stn/1(Out1) -> ik_stn/2(In2)
  In1/1 -> ik_stn/1(In1), n_stn/1(In1)
  ik_stn/1(Out1) -> Out1/1
  In2/1 -> n_stn/2(In2)

== system GPESTN1/STN_cell8/Subsystem/ina ==
  In2 : Inport  Port=1  LatchInput=off
  In1 : Inport  Port=2  LatchInput=off
  h_stn : Subsystem
  ina_stn : Subsystem
  minf : Fcn  Expr=1/(1 + exp(-(u-thetam_stn)/sigmam_stn))
  Out1 : Outport
  wires:
  h_stn/1(Out1) -> ina_stn/3(In3)
  minf/1 -> ina_stn/2(In2)
  In2/1 -> minf/1, h_stn/1(In1), ina_stn/1(In1)
  ina_stn/1(Out1) -> Out1/1
  In1/1 -> h_stn/2(In2)

== system GPESTN1/STN_cell8/Subsystem/it ==
  In2 : Inport  Port=1  LatchInput=off
  In1 : Inport  Port=2  LatchInput=off
  ainf : Fcn  Expr=1/(1 + exp(-(u-thetaa_stn)/sigmaa_stn))
  binf : Fcn  Expr=(1/(1 + exp((u-thetab_stn)/sigmab_stn))) - (1/(1 + exp(-thetab_stn/sigmab_stn)))
  it_stn : Subsystem
  r_stn1 : Subsystem
  Out1 : Outport
  wires:
  ainf/1 -> it_stn/3(In3)
  In2/1 -> r_stn1/1(In1), ainf/1, it_stn/1(In1)
  it_stn/1(Out1) -> Out1/1
  r_stn1/1(Out1) -> binf/1
  binf/1 -> it_stn/2(In2)
  In1/1 -> r_stn1/2(In2)

== system GPESTN1/STN_cell9/Subsystem/iahp ==
  In1 : Inport  Port=1  LatchInput=off
  In2 : Inport  Port=2  LatchInput=off
  In3 : Inport  Port=3  LatchInput=off
  In4 : Inport  Port=4  LatchInput=off
  Fcn : Fcn  Expr=u/(u+k1_stn)
  Fcn1 : Fcn  Expr=(u-ek_stn)*gahp_stn
  Product : Product  SaturateOnIntegerOverflow=on  InputSameDT=on
  Subsystem : Subsystem
  Out1 : Outport
  wires:
  Subsystem/1(Out1) -> Fcn/1
  Fcn1/1 -> Product/2
  Fcn/1 -> Product/1
  In1/1 -> Subsystem/1(In1)
  In2/1 -> Subsystem/2(In2)
  In3/1 -> Fcn1/1
  Product/1 -> Out1/1
  In4/1 -> Subsystem/3(In3)

== system GPESTN1/STN_cell9/Subsystem/ica ==
  In1 : Inport  Orientation=down  Port=1  LatchInput=off
  ica_stn1 : Subsystem
  sinf : Fcn  Expr=1/(1 + exp(-(u-thetas_stn)/sigmas_stn))
  Out1 : Outport
  wires:
  sinf/1 -> ica_stn1/2(In2)
  In1/1 -> sinf/1, ica_stn1/1(In1)
  ica_stn1/1(Out1) -> Out1/1

== system GPESTN1/STN_cell9/Subsystem/ik ==
  In1 : Inport  Port=1  LatchInput=off
  In2 : Inport  Port=2  LatchInput=off
  ik_stn : Subsystem
  n_stn : Subsystem
  Out1 : Outport
  wires:
  n_stn/1(Out1) -> ik_stn/2(In2)
  In1/1 -> ik_stn/1(In1), n_stn/1(In1)
  ik_stn/1(Out1) -> Out1/1
  In2/1 -> n_stn/2(In2)

== system GPESTN1/STN_cell9/Subsystem/ina ==
  In2 : Inport  Port=1  LatchInput=off
  In1 : Inport  Port=2  LatchInput=off
  h_stn : Subsystem
  ina_stn : Subsystem
  minf : Fcn  Expr=1/(1 + exp(-(u-thetam_stn)/sigmam_stn))
  Out1 : Outport
  wires:
  h_stn/1(Out1) -> ina_stn/3(In3)
  minf/1 -> ina_stn/2(In2)
  In2/1 -> minf/1, h_stn/1(In1), ina_stn/1(In1)
  ina_stn/1(Out1) -> Out1/1
  In1/1 -> h_stn/2(In2)

== system GPESTN1/STN_cell9/Subsystem/it ==
  In2 : Inport  Port=1  LatchInput=off
  In1 : Inport  Port=2  LatchInput=off
  ainf : Fcn  Expr=1/(1 + exp(-(u-thetaa_stn)/sigmaa_stn))
  binf : Fcn  Expr=(1/(1 + exp((u-thetab_stn)/sigmab_stn))) - (1/(1 + exp(-thetab_stn/sigmab_stn)))
  it_stn : Subsystem
  r_stn1 : Subsystem
  Out1 : Outport
  wires:
  ainf/1 -> it_stn/3(In3)
  In2/1 -> r_stn1/1(In1), ainf/1, it_stn/1(In1)
  it_stn/1(Out1) -> Out1/1
  r_stn1/1(Out1) -> binf/1
  binf/1 -> it_stn/2(In2)
  In1/1 -> r_stn1/2(In2)

== system GPESTN1/GPE_cell/gpe_cell/iahp/Subsystem ==
  In1 : Inport  Port=1  LatchInput=off
  In2 : Inport  Port=2  LatchInput=off
  In3 : Inport  Port=3  LatchInput=off
  Gain1 : Gain  Gain=epsil_gpe  SaturateOnIntegerOverflow=on
  Gain2 : Gain  Orientation=left  Gain=kca_gpe  SaturateOnIntegerOverflow=on
  Integrator1 : Integrator  InitialConditionSource=external  InitialCondition=cag01
  Scope16 : Scope
      settings: YMin=-80  YMax=60  SaveName=ScopeData3
  Sum1 : Sum  Inputs=---  SaturateOnIntegerOverflow=on  InputSameDT=on
  To Workspace : ToWorkspace  VariableName=cagpe  SampleTime=-1  SaveFormat=Structure
  Out1 : Outport
  wires:
  Sum1/1 -> Gain1/1
  Gain1/1 -> Integrator1/1
  Gain2/1 -> Sum1/3
  Integrator1/1 -> Out1/1, Gain2/1, To Workspace/1, Scope16/1
  In1/1 -> Sum1/1
  In2/1 -> Sum1/2
  In3/1 -> Integrator1/2

== system GPESTN1/GPE_cell/gpe_cell/ica/ica_gpe ==
  In1 : Inport  Port=1  LatchInput=off
  In2 : Inport  Port=2  LatchInput=off
  Fcn1 : Fcn  Expr=u^2*gca_gpe
  Fcn2 : Fcn  Expr=u-eca_gpe
  Product : Product  SaturateOnIntegerOverflow=on  InputSameDT=on
  Out1 : Outport
  wires:
  Fcn1/1 -> Product/2
  Fcn2/1 -> Product/1
  In1/1 -> Fcn2/1
  Product/1 -> Out1/1
  In2/1 -> Fcn1/1

== system GPESTN1/GPE_cell/gpe_cell/ik/ik_gpe ==
  In1 : Inport  Port=1  LatchInput=off
  In2 : Inport  Port=2  LatchInput=off
  Fcn1 : Fcn  Expr=u^4*gk_gpe
  Fcn2 : Fcn  Expr=u-ek_gpe
  Product : Product  SaturateOnIntegerOverflow=on  InputSameDT=on
  Out1 : Outport
  wires:
  Fcn1/1 -> Product/2
  Fcn2/1 -> Product/1
  In1/1 -> Fcn2/1
  Product/1 -> Out1/1
  In2/1 -> Fcn1/1

== system GPESTN1/GPE_cell/gpe_cell/ik/n_gpe ==
  In1 : Inport  Port=1  LatchInput=off
  In2 : Inport  Port=2  LatchInput=off
  1/tau_n : Fcn  Expr=1/(taun0_gpe+ taun1_gpe/(1+exp(-(u-thetataun_gpe)/sigmataun_gpe)))
  Gain : Gain  Gain=phin_gpe  SaturateOnIntegerOverflow=on
  Integrator1 : Integrator  InitialConditionSource=external  InitialCondition=ng01
  Product : Product  SaturateOnIntegerOverflow=on  InputSameDT=on
  Sum1 : Sum  Inputs=|+-  SaturateOnIntegerOverflow=on  InputSameDT=on
  ninf : Fcn  Expr=1/(1 + exp(-(u-thetan_gpe)/sigman_gpe))
  Out1 : Outport
  wires:
  In1/1 -> 1/tau_n/1, ninf/1
  1/tau_n/1 -> Product/1
  Integrator1/1 -> Sum1/2, Out1/1
  ninf/1 -> Sum1/1
  Sum1/1 -> Product/2
  Product/1 -> Gain/1
  Gain/1 -> Integrator1/1
  In2/1 -> Integrator1/2

== system GPESTN1/GPE_cell/gpe_cell/ina/h_gpe ==
  In1 : Inport  Port=1  LatchInput=off
  In2 : Inport  Port=2  LatchInput=off
  1/tau_h : Fcn  Expr=1/(tauh0_gpe + tauh1_gpe/(1+exp(-(u-thetatauh_gpe)/sigmatauh_gpe)))
  Gain : Gain  Gain=phih_gpe  SaturateOnIntegerOverflow=on
  Integrator1 : Integrator  InitialConditionSource=external  InitialCondition=hg01
  Product : Product  SaturateOnIntegerOverflow=on  InputSameDT=on
  Sum1 : Sum  Inputs=|+-  SaturateOnIntegerOverflow=on  InputSameDT=on
  hinf : Fcn  Expr=1/(1 + exp(-(u-thetah_gpe)/sigmah_gpe))
  Out1 : Outport
  wires:
  In1/1 -> 1/tau_h/1, hinf/1
  1/tau_h/1 -> Product/1
  Integrator1/1 -> Sum1/2, Out1/1
  hinf/1 -> Sum1/1
  Sum1/1 -> Product/2
  Product/1 -> Gain/1
  Gain/1 -> Integrator1/1
  In2/1 -> Integrator1/2

== system GPESTN1/GPE_cell/gpe_cell/ina/ina_gpe ==
  In1 : Inport  Port=1  LatchInput=off
  In2 : Inport  Port=2  LatchInput=off
  In3 : Inport  Port=3  LatchInput=off
  Fcn1 : Fcn  Expr=u^3*gna_gpe
  Fcn2 : Fcn  Expr=u-ena_gpe
  Product : Product  Inputs=3  SaturateOnIntegerOverflow=on  InputSameDT=on
  Out1 : Outport
  wires:
  Fcn1/1 -> Product/2
  Fcn2/1 -> Product/1
  In1/1 -> Fcn2/1
  Product/1 -> Out1/1
  In3/1 -> Product/3
  In2/1 -> Fcn1/1

== system GPESTN1/GPE_cell/gpe_cell/it/it_gpe ==
  In1 : Inport  Port=1  LatchInput=off
  In2 : Inport  Port=2  LatchInput=off
  In3 : Inport  Port=3  LatchInput=off
  Fcn1 : Fcn  Expr=u^2*gt_gpe
  Fcn2 : Fcn  Expr=u-eca_gpe
  Fcn3 : Fcn  Expr=u^3
  Product : Product  Inputs=3  SaturateOnIntegerOverflow=on  InputSameDT=on
  Out1 : Outport
  wires:
  Fcn1/1 -> Product/2
  Fcn2/1 -> Product/1
  In1/1 -> Fcn2/1
  Product/1 -> Out1/1
  In2/1 -> Fcn1/1
  In3/1 -> Fcn3/1
  Fcn3/1 -> Product/3

== system GPESTN1/GPE_cell/gpe_cell/it/r_gpe ==
  In1 : Inport  Port=1  LatchInput=off
  In2 : Inport  Port=2  LatchInput=off
  1/tau_r : Fcn  Expr=1/taur_gpe
  Gain : Gain  Gain=phir_gpe  SaturateOnIntegerOverflow=on
  Integrator1 : Integrator  InitialConditionSource=external  InitialCondition=rg01
  Product : Product  SaturateOnIntegerOverflow=on  InputSameDT=on
  Sum1 : Sum  Inputs=|+-  SaturateOnIntegerOverflow=on  InputSameDT=on
  rinf : Fcn  Expr=1/(1 + exp(-(u-thetar_gpe)/sigmar_gpe))
  Out1 : Outport
  wires:
  In1/1 -> 1/tau_r/1, rinf/1
  1/tau_r/1 -> Product/1
  Integrator1/1 -> Sum1/2, Out1/1
  rinf/1 -> Sum1/1
  Sum1/1 -> Product/2
  Product/1 -> Gain/1
  Gain/1 -> Integrator1/1
  In2/1 -> Integrator1/2

== system GPESTN1/GPE_cell1/gpe_cell/iahp/Subsystem ==
  In1 : Inport  Port=1  LatchInput=off
  In2 : Inport  Port=2  LatchInput=off
  In3 : Inport  Port=3  LatchInput=off
  Gain1 : Gain  Gain=epsil_gpe  SaturateOnIntegerOverflow=on
  Gain2 : Gain  Orientation=left  Gain=kca_gpe  SaturateOnIntegerOverflow=on
  Integrator1 : Integrator  InitialConditionSource=external  InitialCondition=cag01
  Sum1 : Sum  Inputs=---  SaturateOnIntegerOverflow=on  InputSameDT=on
  Out1 : Outport
  wires:
  Sum1/1 -> Gain1/1
  Gain1/1 -> Integrator1/1
  Gain2/1 -> Sum1/3
  Integrator1/1 -> Out1/1, Gain2/1
  In1/1 -> Sum1/1
  In2/1 -> Sum1/2
  In3/1 -> Integrator1/2

== system GPESTN1/GPE_cell1/gpe_cell/ica/ica_gpe ==
  In1 : Inport  Port=1  LatchInput=off
  In2 : Inport  Port=2  LatchInput=off
  Fcn1 : Fcn  Expr=u^2*gca_gpe
  Fcn2 : Fcn  Expr=u-eca_gpe
  Product : Product  SaturateOnIntegerOverflow=on  InputSameDT=on
  Out1 : Outport
  wires:
  Fcn1/1 -> Product/2
  Fcn2/1 -> Product/1
  In1/1 -> Fcn2/1
  Product/1 -> Out1/1
  In2/1 -> Fcn1/1

== system GPESTN1/GPE_cell1/gpe_cell/ik/ik_gpe ==
  In1 : Inport  Port=1  LatchInput=off
  In2 : Inport  Port=2  LatchInput=off
  Fcn1 : Fcn  Expr=u^4*gk_gpe
  Fcn2 : Fcn  Expr=u-ek_gpe
  Product : Product  SaturateOnIntegerOverflow=on  InputSameDT=on
  Out1 : Outport
  wires:
  Fcn1/1 -> Product/2
  Fcn2/1 -> Product/1
  In1/1 -> Fcn2/1
  Product/1 -> Out1/1
  In2/1 -> Fcn1/1

== system GPESTN1/GPE_cell1/gpe_cell/ik/n_gpe ==
  In1 : Inport  Port=1  LatchInput=off
  In2 : Inport  Port=2  LatchInput=off
  1/tau_n : Fcn  Expr=1/(taun0_gpe+ taun1_gpe/(1+exp(-(u-thetataun_gpe)/sigmataun_gpe)))
  Gain : Gain  Gain=phin_gpe  SaturateOnIntegerOverflow=on
  Integrator1 : Integrator  InitialConditionSource=external  InitialCondition=ng01
  Product : Product  SaturateOnIntegerOverflow=on  InputSameDT=on
  Sum1 : Sum  Inputs=|+-  SaturateOnIntegerOverflow=on  InputSameDT=on
  ninf : Fcn  Expr=1/(1 + exp(-(u-thetan_gpe)/sigman_gpe))
  Out1 : Outport
  wires:
  In1/1 -> 1/tau_n/1, ninf/1
  1/tau_n/1 -> Product/1
  Integrator1/1 -> Sum1/2, Out1/1
  ninf/1 -> Sum1/1
  Sum1/1 -> Product/2
  Product/1 -> Gain/1
  Gain/1 -> Integrator1/1
  In2/1 -> Integrator1/2

== system GPESTN1/GPE_cell1/gpe_cell/ina/h_gpe ==
  In1 : Inport  Port=1  LatchInput=off
  In2 : Inport  Port=2  LatchInput=off
  1/tau_h : Fcn  Expr=1/(tauh0_gpe + tauh1_gpe/(1+exp(-(u-thetatauh_gpe)/sigmatauh_gpe)))
  Gain : Gain  Gain=phih_gpe  SaturateOnIntegerOverflow=on
  Integrator1 : Integrator  InitialConditionSource=external  InitialCondition=hg01
  Product : Product  SaturateOnIntegerOverflow=on  InputSameDT=on
  Sum1 : Sum  Inputs=|+-  SaturateOnIntegerOverflow=on  InputSameDT=on
  hinf : Fcn  Expr=1/(1 + exp(-(u-thetah_gpe)/sigmah_gpe))
  Out1 : Outport
  wires:
  In1/1 -> 1/tau_h/1, hinf/1
  1/tau_h/1 -> Product/1
  Integrator1/1 -> Sum1/2, Out1/1
  hinf/1 -> Sum1/1
  Sum1/1 -> Product/2
  Product/1 -> Gain/1
  Gain/1 -> Integrator1/1
  In2/1 -> Integrator1/2

== system GPESTN1/GPE_cell1/gpe_cell/ina/ina_gpe ==
  In1 : Inport  Port=1  LatchInput=off
  In2 : Inport  Port=2  LatchInput=off
  In3 : Inport  Port=3  LatchInput=off
  Fcn1 : Fcn  Expr=u^3*gna_gpe
  Fcn2 : Fcn  Expr=u-ena_gpe
  Product : Product  Inputs=3  SaturateOnIntegerOverflow=on  InputSameDT=on
  Out1 : Outport
  wires:
  Fcn1/1 -> Product/2
  Fcn2/1 -> Product/1
  In1/1 -> Fcn2/1
  Product/1 -> Out1/1
  In3/1 -> Product/3
  In2/1 -> Fcn1/1

== system GPESTN1/GPE_cell1/gpe_cell/it/it_gpe ==
  In1 : Inport  Port=1  LatchInput=off
  In2 : Inport  Port=2  LatchInput=off
  In3 : Inport  Port=3  LatchInput=off
  Fcn1 : Fcn  Expr=u^2*gt_gpe
  Fcn2 : Fcn  Expr=u-eca_gpe
  Fcn3 : Fcn  Expr=u^3
  Product : Product  Inputs=3  SaturateOnIntegerOverflow=on  InputSameDT=on
  Out1 : Outport
  wires:
  Fcn1/1 -> Product/2
  Fcn2/1 -> Product/1
  In1/1 -> Fcn2/1
  Product/1 -> Out1/1
  In2/1 -> Fcn1/1
  In3/1 -> Fcn3/1
  Fcn3/1 -> Product/3

== system GPESTN1/GPE_cell1/gpe_cell/it/r_gpe ==
  In1 : Inport  Port=1  LatchInput=off
  In2 : Inport  Port=2  LatchInput=off
  1/tau_r : Fcn  Expr=1/taur_gpe
  Gain : Gain  Gain=phir_gpe  SaturateOnIntegerOverflow=on
  Integrator1 : Integrator  InitialConditionSource=external  InitialCondition=rg01
  Product : Product  SaturateOnIntegerOverflow=on  InputSameDT=on
  Sum1 : Sum  Inputs=|+-  SaturateOnIntegerOverflow=on  InputSameDT=on
  rinf : Fcn  Expr=1/(1 + exp(-(u-thetar_gpe)/sigmar_gpe))
  Out1 : Outport
  wires:
  In1/1 -> 1/tau_r/1, rinf/1
  1/tau_r/1 -> Product/1
  Integrator1/1 -> Sum1/2, Out1/1
  rinf/1 -> Sum1/1
  Sum1/1 -> Product/2
  Product/1 -> Gain/1
  Gain/1 -> Integrator1/1
  In2/1 -> Integrator1/2

== system GPESTN1/GPE_cell10/gpe_cell/iahp/Subsystem ==
  In1 : Inport  Port=1  LatchInput=off
  In2 : Inport  Port=2  LatchInput=off
  In3 : Inport  Port=3  LatchInput=off
  Gain1 : Gain  Gain=epsil_gpe  SaturateOnIntegerOverflow=on
  Gain2 : Gain  Orientation=left  Gain=kca_gpe  SaturateOnIntegerOverflow=on
  Integrator1 : Integrator  InitialConditionSource=external  InitialCondition=cag01
  Sum1 : Sum  Inputs=---  SaturateOnIntegerOverflow=on  InputSameDT=on
  Out1 : Outport
  wires:
  Sum1/1 -> Gain1/1
  Gain1/1 -> Integrator1/1
  Gain2/1 -> Sum1/3
  Integrator1/1 -> Out1/1, Gain2/1
  In1/1 -> Sum1/1
  In2/1 -> Sum1/2
  In3/1 -> Integrator1/2

== system GPESTN1/GPE_cell10/gpe_cell/ica/ica_gpe ==
  In1 : Inport  Port=1  LatchInput=off
  In2 : Inport  Port=2  LatchInput=off
  Fcn1 : Fcn  Expr=u^2*gca_gpe
  Fcn2 : Fcn  Expr=u-eca_gpe
  Product : Product  SaturateOnIntegerOverflow=on  InputSameDT=on
  Out1 : Outport
  wires:
  Fcn1/1 -> Product/2
  Fcn2/1 -> Product/1
  In1/1 -> Fcn2/1
  Product/1 -> Out1/1
  In2/1 -> Fcn1/1

== system GPESTN1/GPE_cell10/gpe_cell/ik/ik_gpe ==
  In1 : Inport  Port=1  LatchInput=off
  In2 : Inport  Port=2  LatchInput=off
  Fcn1 : Fcn  Expr=u^4*gk_gpe
  Fcn2 : Fcn  Expr=u-ek_gpe
  Product : Product  SaturateOnIntegerOverflow=on  InputSameDT=on
  Out1 : Outport
  wires:
  Fcn1/1 -> Product/2
  Fcn2/1 -> Product/1
  In1/1 -> Fcn2/1
  Product/1 -> Out1/1
  In2/1 -> Fcn1/1

== system GPESTN1/GPE_cell10/gpe_cell/ik/n_gpe ==
  In1 : Inport  Port=1  LatchInput=off
  In2 : Inport  Port=2  LatchInput=off
  1/tau_n : Fcn  Expr=1/(taun0_gpe+ taun1_gpe/(1+exp(-(u-thetataun_gpe)/sigmataun_gpe)))
  Gain : Gain  Gain=phin_gpe  SaturateOnIntegerOverflow=on
  Integrator1 : Integrator  InitialConditionSource=external  InitialCondition=ng01
  Product : Product  SaturateOnIntegerOverflow=on  InputSameDT=on
  Sum1 : Sum  Inputs=|+-  SaturateOnIntegerOverflow=on  InputSameDT=on
  ninf : Fcn  Expr=1/(1 + exp(-(u-thetan_gpe)/sigman_gpe))
  Out1 : Outport
  wires:
  In1/1 -> 1/tau_n/1, ninf/1
  1/tau_n/1 -> Product/1
  Integrator1/1 -> Sum1/2, Out1/1
  ninf/1 -> Sum1/1
  Sum1/1 -> Product/2
  Product/1 -> Gain/1
  Gain/1 -> Integrator1/1
  In2/1 -> Integrator1/2

== system GPESTN1/GPE_cell10/gpe_cell/ina/h_gpe ==
  In1 : Inport  Port=1  LatchInput=off
  In2 : Inport  Port=2  LatchInput=off
  1/tau_h : Fcn  Expr=1/(tauh0_gpe + tauh1_gpe/(1+exp(-(u-thetatauh_gpe)/sigmatauh_gpe)))
  Gain : Gain  Gain=phih_gpe  SaturateOnIntegerOverflow=on
  Integrator1 : Integrator  InitialConditionSource=external  InitialCondition=hg01
  Product : Product  SaturateOnIntegerOverflow=on  InputSameDT=on
  Sum1 : Sum  Inputs=|+-  SaturateOnIntegerOverflow=on  InputSameDT=on
  hinf : Fcn  Expr=1/(1 + exp(-(u-thetah_gpe)/sigmah_gpe))
  Out1 : Outport
  wires:
  In1/1 -> 1/tau_h/1, hinf/1
  1/tau_h/1 -> Product/1
  Integrator1/1 -> Sum1/2, Out1/1
  hinf/1 -> Sum1/1
  Sum1/1 -> Product/2
  Product/1 -> Gain/1
  Gain/1 -> Integrator1/1
  In2/1 -> Integrator1/2

== system GPESTN1/GPE_cell10/gpe_cell/ina/ina_gpe ==
  In1 : Inport  Port=1  LatchInput=off
  In2 : Inport  Port=2  LatchInput=off
  In3 : Inport  Port=3  LatchInput=off
  Fcn1 : Fcn  Expr=u^3*gna_gpe
  Fcn2 : Fcn  Expr=u-ena_gpe
  Product : Product  Inputs=3  SaturateOnIntegerOverflow=on  InputSameDT=on
  Out1 : Outport
  wires:
  Fcn1/1 -> Product/2
  Fcn2/1 -> Product/1
  In1/1 -> Fcn2/1
  Product/1 -> Out1/1
  In3/1 -> Product/3
  In2/1 -> Fcn1/1

== system GPESTN1/GPE_cell10/gpe_cell/it/it_gpe ==
  In1 : Inport  Port=1  LatchInput=off
  In2 : Inport  Port=2  LatchInput=off
  In3 : Inport  Port=3  LatchInput=off
  Fcn1 : Fcn  Expr=u^2*gt_gpe
  Fcn2 : Fcn  Expr=u-eca_gpe
  Fcn3 : Fcn  Expr=u^3
  Product : Product  Inputs=3  SaturateOnIntegerOverflow=on  InputSameDT=on
  Out1 : Outport
  wires:
  Fcn1/1 -> Product/2
  Fcn2/1 -> Product/1
  In1/1 -> Fcn2/1
  Product/1 -> Out1/1
  In2/1 -> Fcn1/1
  In3/1 -> Fcn3/1
  Fcn3/1 -> Product/3

== system GPESTN1/GPE_cell10/gpe_cell/it/r_gpe ==
  In1 : Inport  Port=1  LatchInput=off
  In2 : Inport  Port=2  LatchInput=off
  1/tau_r : Fcn  Expr=1/taur_gpe
  Gain : Gain  Gain=phir_gpe  SaturateOnIntegerOverflow=on
  Integrator1 : Integrator  InitialConditionSource=external  InitialCondition=rg01
  Product : Product  SaturateOnIntegerOverflow=on  InputSameDT=on
  Sum1 : Sum  Inputs=|+-  SaturateOnIntegerOverflow=on  InputSameDT=on
  rinf : Fcn  Expr=1/(1 + exp(-(u-thetar_gpe)/sigmar_gpe))
  Out1 : Outport
  wires:
  In1/1 -> 1/tau_r/1, rinf/1
  1/tau_r/1 -> Product/1
  Integrator1/1 -> Sum1/2, Out1/1
  rinf/1 -> Sum1/1
  Sum1/1 -> Product/2
  Product/1 -> Gain/1
  Gain/1 -> Integrator1/1
  In2/1 -> Integrator1/2
